simulink model "extControlwithTCP"  (R2019a)
settings: Solver=FixedStepAuto  StartTime=0.0  StopTime=501  FixedStep=0.01  RelTol=1e-3
PreLoadFcn:
  | load('tumbleweed_constants.mat')
InitFcn:
  | coder.extrinsic('controlsolver')
undefined symbols (not defined in the file): d, f, g, Ixx, Iyy, Izz, m, maxr, mf, minr, mu0, R, v_thres, vmax, YY
libraries: instrumentlib x2, simulink x1
settings Model: EnablePacing=on  Creator=racha  LastModifiedBy=racha
settings RTWCC: TargetLang=C++
settings GRTTargetCC: TargetLangStandard=C++03 (ISO)  MultiInstanceERTCode=on  CodeInterfacePackaging=C++ class

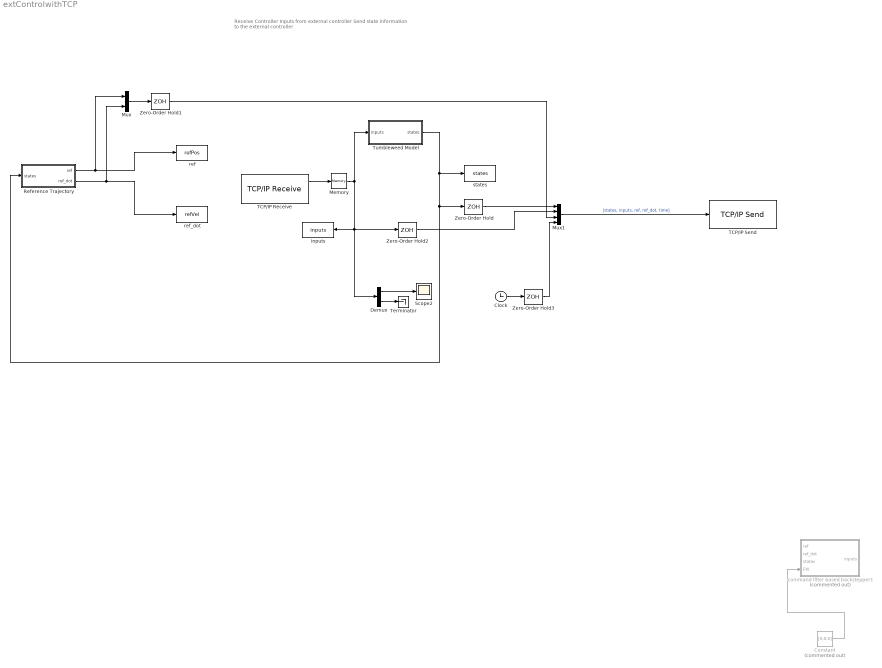
== system extControlwithTCP ==
  note: Receive Controller Inputs from external controller
      | Send state information to the external controller
  Clock : Clock
  Constant : Constant  Commented=on  Value=[0;0;0]
  Demux : Demux  Outputs=[1;17]
  Memory : Memory  InitialCondition=[d/2;-d/2;d/2;-d/2;d/2;-d/2;zeros(12,1)]
  Mux : Mux  Inputs=[3;3]
  Mux1 : Mux  Inputs=[13;18;6;1]
  Reference Trajectory : Subsystem
  Scope2 : Scope
  TCP/IP Receive : instrumentlib/TCP//IP Receive  Priority=4  Host=localhost  Port=54330  DataSize="[18   1]"  EnableBlockingMode=off  Timeout=10  SampleTime=0.01  DataType=double  ByteOrder=LittleEndian  ASCIIFormatting=%f,  Terminator=LF
      settings: SourceProductName=Instrument Control Toolbox
  TCP/IP Send : instrumentlib/TCP//IP Send  Priority=1  Host=localhost  Port=54320  EnableBlockingMode=off  Timeout=10  ByteOrder=LittleEndian  TransferDelay=off
      settings: SourceProductName=Instrument Control Toolbox
  Terminator : Terminator
  Tumbleweed Model : Subsystem
  Zero-Order Hold{,1..3} (4 alike) : ZeroOrderHold  SampleTime=0.01
  command filter based backstepper1 : Subsystem  Commented=on
  inputs : ToWorkspace  VariableName=inputs  SampleTime=-1
      settings: Save2DSignal=2-D array (concatenate along first dimension)
  ref : ToWorkspace  VariableName=refPos  SampleTime=-1
      settings: Save2DSignal=2-D array (concatenate along first dimension)
  ref_dot : ToWorkspace  VariableName=refVel  SampleTime=-1
      settings: Save2DSignal=2-D array (concatenate along first dimension)
  states : ToWorkspace  VariableName=states  SampleTime=-1
      settings: Save2DSignal=2-D array (concatenate along first dimension)
  wires:
  Reference Trajectory/1(ref) -> Mux/1, ref/1
  Reference Trajectory/2("ref_dot ") -> Mux/2, ref_dot/1
  Constant/1 -> command filter based backstepper1/4(FW)
  TCP/IP Receive/1 -> Memory/1
  Mux/1 -> Zero-Order Hold1/1
  Tumbleweed Model/1("states ") -> Reference Trajectory/1(states), Zero-Order Hold/1, states/1
  Zero-Order Hold1/1 -> Mux1/3
  Memory/1 -> Demux/1, inputs/1, Zero-Order Hold2/1, Tumbleweed Model/1(inputs)
  Demux/1 -> Scope2/1
  Demux/2 -> Terminator/1
  Zero-Order Hold/1 -> Mux1/1
  Mux1/1 -> TCP/IP Send/1  "[states, inputs, ref, ref_dot, time]"
  Zero-Order Hold2/1 -> Mux1/2
  Clock/1 -> Zero-Order Hold3/1
  Zero-Order Hold3/1 -> Mux1/4

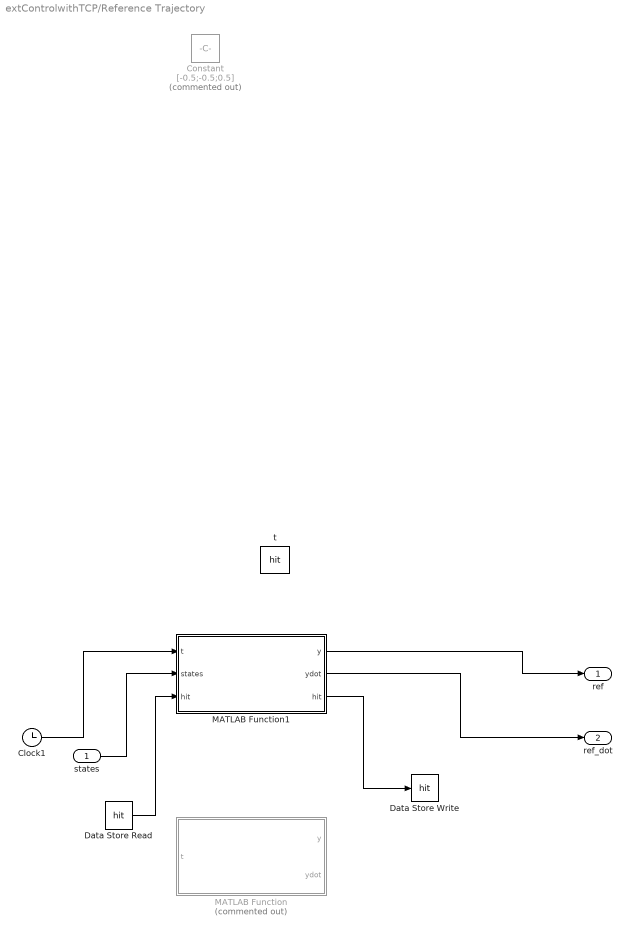
== system extControlwithTCP/Reference Trajectory ==
  states : Inport
  Clock1 : Clock
  Constant : Constant  Commented=on  Value=[-0.5;-0.5;0.5]
  Data Store Read : DataStoreRead  DataStoreName=hit
  Data Store Write : DataStoreWrite  DataStoreName=hit
  MATLAB Function : MATLAB Function  Commented=on  TreatAsAtomicUnit=on
  MATLAB Function1 : MATLAB Function  TreatAsAtomicUnit=on
  t : DataStoreMemory  DataStoreName=hit  ReadBeforeWriteMsg=warning  WriteAfterWriteMsg=warning  WriteAfterReadMsg=warning  ShowAdditionalParam=off
  ref : Outport
  "ref_dot " : Outport  Port=2
  wires:
  MATLAB Function1/2(ydot) -> "ref_dot "/1
  Data Store Read/1 -> MATLAB Function1/3("hit ")
  states/1 -> MATLAB Function1/2(states)
  Clock1/1 -> MATLAB Function1/1(t)
  MATLAB Function1/3(hit) -> Data Store Write/1
  MATLAB Function1/1(y) -> ref/1

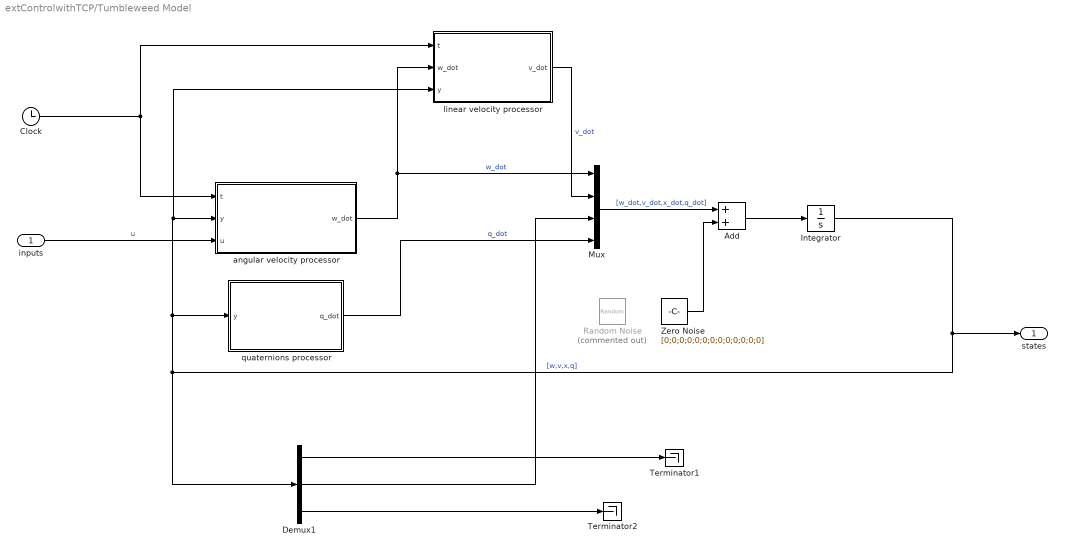
== system extControlwithTCP/Tumbleweed Model ==
  inputs : Inport
  Add : Sum
  Clock : Clock
  Demux1 : Demux  Outputs=[3;3;7]
  Integrator : Integrator  InitialCondition=|
      | [0;
      | 0.001; 0; 0.0005; 0; 0;0;0;R;1;0;0;0]
  Mux : Mux  Inputs=[3;3;3;4]
  Random Noise : RandomNumber  Commented=on  Mean=zeros(13,1)  Variance=[0.1;0.1;0.1;0.1;0.1;0;0.1;0.1;0;0.01;0.01;0.01;0.01]  SampleTime=0.001
  Terminator1 : Terminator
  Terminator2 : Terminator
  Zero Noise : Constant  Value=[0;0;0;0;0;0;0;0;0;0;0;0;0]  OutDataTypeStr=Inherit: Inherit via back propagation
  angular velocity processor : MATLAB Function  TreatAsAtomicUnit=on
  linear velocity processor : MATLAB Function  TreatAsAtomicUnit=on
  quaternions processor : MATLAB Function  TreatAsAtomicUnit=on
  "states " : Outport
  wires:
  Clock/1 -> linear velocity processor/1(t), angular velocity processor/1(t)
  angular velocity processor/1(w_dot) -> Mux/1, linear velocity processor/2(w_dot)  "w_dot"
  quaternions processor/1(q_dot) -> Mux/4  "q_dot"
  inputs/1 -> angular velocity processor/3(u)  "u"
  linear velocity processor/1(v_dot) -> Mux/2  "v_dot"
  Demux1/1 -> Terminator1/1
  Demux1/2 -> Mux/3
  Integrator/1 -> Demux1/1, linear velocity processor/3(y), angular velocity processor/2(y), quaternions processor/1(y), "states "/1  "[w,v,x,q]"
  Demux1/3 -> Terminator2/1
  Mux/1 -> Add/1  "[w_dot,v_dot,x_dot,q_dot]"
  Add/1 -> Integrator/1
  Zero Noise/1 -> Add/2

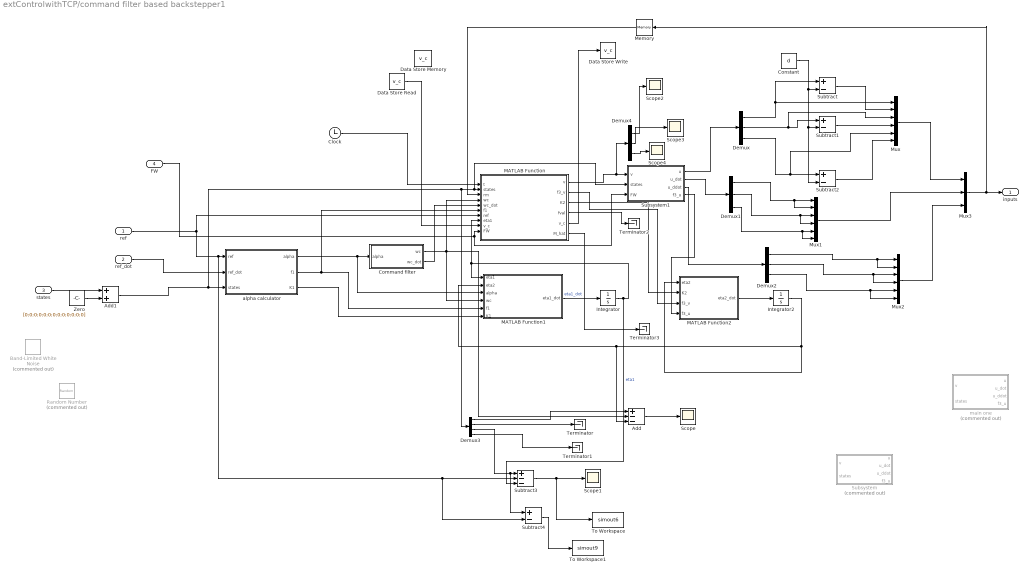
== system extControlwithTCP/command filter based backstepper1 ==
  ref : Inport
  "ref_dot " : Inport  Port=2
  states : Inport  Port=3
  FW : Inport  Port=4
  Add : Sum  Inputs=+--
  Add1 : Sum
  Band-Limited White Noise : simulink/Sources/Band-Limited White Noise  Commented=on  Cov=[0.002;0.002;0.002;0.002;0.002;0.001;0.05;0.05;0.05;0.001;0.001;0.001;0.001]  Ts=0.001  seed=[23340]
  Clock : Clock
  Command filter : Subsystem
  Constant : Constant  Value=d
  Data Store Memory : DataStoreMemory  DataStoreName=v_c  ReadBeforeWriteMsg=warning  WriteAfterWriteMsg=warning  WriteAfterReadMsg=warning  InitialValue=[0.325;0.325;0.325;0]  ShowAdditionalParam=off
  Data Store Read : DataStoreRead  DataStoreName=v_c
  Data Store Write : DataStoreWrite  DataStoreName=v_c
  Demux{,1..2,4} (4 alike) : Demux  Outputs=3
  Demux3 : Demux  Outputs=[3;3;3;4]
  Integrator : Integrator  InitialCondition=[0;0;0]
  Integrator2 : Integrator  InitialCondition=[0;0;0]
  MATLAB Function : MATLAB Function  TreatAsAtomicUnit=on
  MATLAB Function1 : MATLAB Function  TreatAsAtomicUnit=on
  MATLAB Function2 : MATLAB Function  TreatAsAtomicUnit=on
  Memory : Memory  InitialCondition=[d/2;-d/2;d/2;-d/2;d/2;-d/2;0;0;0;0;0;0;0;0;0;0;0;0]
  Mux : Mux  Inputs=6
  Mux1 : Mux  Inputs=6
  Mux2 : Mux  Inputs=6
  Mux3 : Mux  Inputs=3
  Random Number : RandomNumber  Commented=on  Mean=zeros(13,1)  Variance=[0.1;0.1;0.1;0.1;0.1;0.1;0.2;0.2;0.2;0.01;0.01;0.01;0.01]  Seed=randi(1000,13,1)  SampleTime=0.001
  Scope{,1..4} (5 alike) : Scope
  Subsystem : Subsystem  Commented=on
  Subsystem1 : Subsystem
  Subtract{,1..2,4} (4 alike) : Sum  Inputs=+-
  Subtract3 : Sum  Inputs=+--
  Terminator{,1..3} (4 alike) : Terminator
  To Workspace : ToWorkspace  VariableName=simout6  SaveFormat=Timeseries  SampleTime=-1
  To Workspace1 : ToWorkspace  VariableName=simout9  SaveFormat=Timeseries  SampleTime=-1
  Zero : Constant  Value=[0;0;0;0;0;0;0;0;0;0;0;0;0]  OutDataTypeStr=Inherit: Inherit via back propagation
  alpha calculator : MATLAB Function  TreatAsAtomicUnit=on
  main one : Subsystem  Commented=on
  inputs : Outport
  wires:
  alpha calculator/1(alpha) -> Command filter/1(alpha), MATLAB Function1/3(alpha)
  MATLAB Function1/1(eta1_dot) -> Integrator/1  "eta1_dot"
  Integrator/1 -> Subtract3/3, MATLAB Function/8(eta1), MATLAB Function1/1(eta1)  "eta1"
  alpha calculator/2(f1) -> MATLAB Function/6(f1), MATLAB Function1/5(f1)
  alpha calculator/3(K1) -> MATLAB Function1/6(K1)
  ref/1 -> MATLAB Function/7(ref), Subtract4/2, Subtract3/2, alpha calculator/1(ref)
  "ref_dot "/1 -> alpha calculator/2(ref_dot)
  Command filter/2(wc_dot) -> MATLAB Function/5(wc_dot)
  Command filter/1(wc) -> MATLAB Function/4(wc), MATLAB Function1/4(wc), Add/2
  MATLAB Function/1(v) -> Demux4/1, Subsystem1/1(v)
  Subsystem1/1(u) -> Demux/1
  Subsystem1/2(u_dot) -> Demux1/1
  Mux3/1 -> Memory/1, inputs/1
  MATLAB Function/3(K2) -> MATLAB Function2/2(K2)
  MATLAB Function/2(f3_v) -> MATLAB Function2/3(f3_v)
  Subsystem1/4(f3_u) -> MATLAB Function2/4(f3_u)
  MATLAB Function2/1(eta2_dot) -> Integrator2/1
  Integrator2/1 -> MATLAB Function1/2(eta2), Add/3, MATLAB Function2/1(eta2)
  Subsystem1/3(u_ddot) -> Demux2/1
  Demux/3 -> Mux/5, Subtract2/1
  Demux/2 -> Mux/3, Subtract1/1
  Demux/1 -> Mux/1, Subtract/1
  Constant/1 -> Subtract2/2, Subtract1/2, Subtract/2
  Subtract/1 -> Mux/2
  Subtract1/1 -> Mux/4
  Subtract2/1 -> Mux/6
  Mux/1 -> Mux3/1
  Demux1/1 -> Mux1/2, Mux1/1
  Demux1/2 -> Mux1/4, Mux1/3
  Demux1/3 -> Mux1/6, Mux1/5
  Demux2/3 -> Mux2/6, Mux2/5
  Demux2/1 -> Mux2/2, Mux2/1
  Demux2/2 -> Mux2/4, Mux2/3
  Mux1/1 -> Mux3/2
  Mux2/1 -> Mux3/3
  Memory/1 -> MATLAB Function/3(rm)
  Clock/1 -> MATLAB Function/1(t)
  MATLAB Function/4(fval) -> Terminator2/1
  Data Store Read/1 -> MATLAB Function/9("v_c ")
  MATLAB Function/5(v_c) -> Data Store Write/1
  MATLAB Function/6(M_hat) -> Terminator3/1
  Demux3/2 -> Terminator/1
  Demux3/1 -> Add/1
  Add/1 -> Scope/1
  Demux3/4 -> Terminator1/1
  Demux3/3 -> Subtract4/1, Subtract3/1
  Subtract3/1 -> To Workspace/1, Scope1/1
  Add1/1 -> Demux3/1, Subsystem1/2(states), MATLAB Function/2(states), alpha calculator/3(states)
  states/1 -> Add1/1
  Zero/1 -> Add1/2
  FW/1 -> Subsystem1/3(FW), MATLAB Function/10(FW)
  Subtract4/1 -> To Workspace1/1
  Demux4/1 -> Scope2/1
  Demux4/2 -> Scope3/1
  Demux4/3 -> Scope4/1

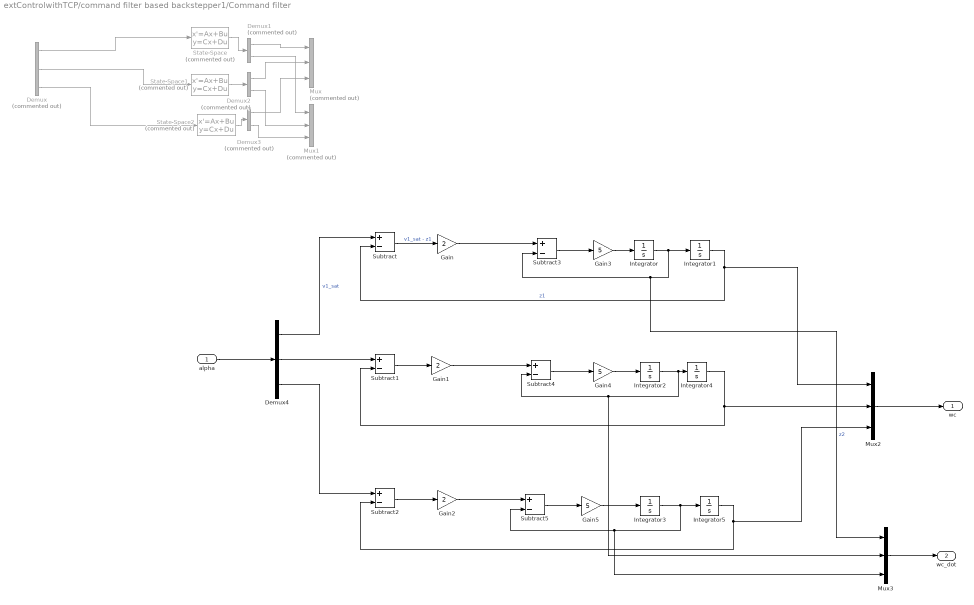
== system extControlwithTCP/command filter based backstepper1/Command filter ==
  alpha : Inport
  Demux : Demux  Commented=on  Outputs=3
  Demux1 : Demux  Commented=on  Outputs=2
  Demux2 : Demux  Commented=on  Outputs=2
  Demux3 : Demux  Commented=on  Outputs=2
  Demux4 : Demux  Outputs=3
  Gain : Gain  Gain=2
  Gain1 : Gain  Gain=2
  Gain2 : Gain  Gain=2
  Gain3 : Gain  Gain=5
  Gain4 : Gain  Gain=5
  Gain5 : Gain  Gain=5
  Integrator{,1..5} (6 alike) : Integrator
  Mux : Mux  Commented=on  Inputs=3
  Mux1 : Mux  Commented=on  Inputs=3
  Mux2 : Mux  Inputs=3
  Mux3 : Mux  Inputs=3
  State-Space : StateSpace  Commented=on  A=[0, 10; -2*0.8*10, -10]  B=[0;20]  C=[1,0;0,1]  D=[0;0]  InitialCondition=[0;0]
  State-Space1 : StateSpace  Commented=on  A=[0, 10; -2*0.8*10, -10]  B=[0;20]  C=[1,0;0,1]  D=[0;0]  InitialCondition=[0;0]
  State-Space2 : StateSpace  Commented=on  A=[0, 10; -2*0.8*10, -10]  B=[0;5]  C=[1,0;0,1]  D=[0;0]  InitialCondition=[0;0]
  Subtract{,1..5} (6 alike) : Sum  Inputs=+-
  wc : Outport
  wc_dot : Outport  Port=2
  wires:
  State-Space/1 -> Demux1/1
  Demux/1 -> State-Space/1
  Demux/2 -> State-Space1/1
  Demux/3 -> State-Space2/1
  State-Space1/1 -> Demux2/1
  Demux2/1 -> Mux/2
  State-Space2/1 -> Demux3/1
  Demux1/1 -> Mux/1
  Demux3/1 -> Mux/3
  Demux1/2 -> Mux1/1
  Demux2/2 -> Mux1/2
  Demux3/2 -> Mux1/3
  Mux2/1 -> wc/1
  alpha/1 -> Demux4/1
  Demux4/1 -> Subtract/1  "v1_sat"
  Gain3/1 -> Integrator/1
  Subtract/1 -> Gain/1  "v1_sat - z1"
  Subtract5/1 -> Gain5/1
  Gain/1 -> Subtract3/1
  Subtract2/1 -> Gain2/1
  Integrator2/1 -> Mux3/2, Subtract4/2, Integrator4/1
  Gain4/1 -> Integrator2/1
  Subtract1/1 -> Gain1/1
  Subtract3/1 -> Gain3/1
  Subtract4/1 -> Gain4/1
  Gain5/1 -> Integrator3/1
  Integrator/1 -> Integrator1/1, Mux3/1, Subtract3/2  "z2"
  Integrator5/1 -> Subtract2/2, Mux2/3
  Mux3/1 -> wc_dot/1
  Gain1/1 -> Subtract4/1
  Gain2/1 -> Subtract5/1
  Integrator4/1 -> Subtract1/2, Mux2/2
  Integrator3/1 -> Mux3/3, Subtract5/2, Integrator5/1
  Integrator1/1 -> Subtract/2, Mux2/1  "z1"
  Demux4/2 -> Subtract1/1
  Demux4/3 -> Subtract2/1

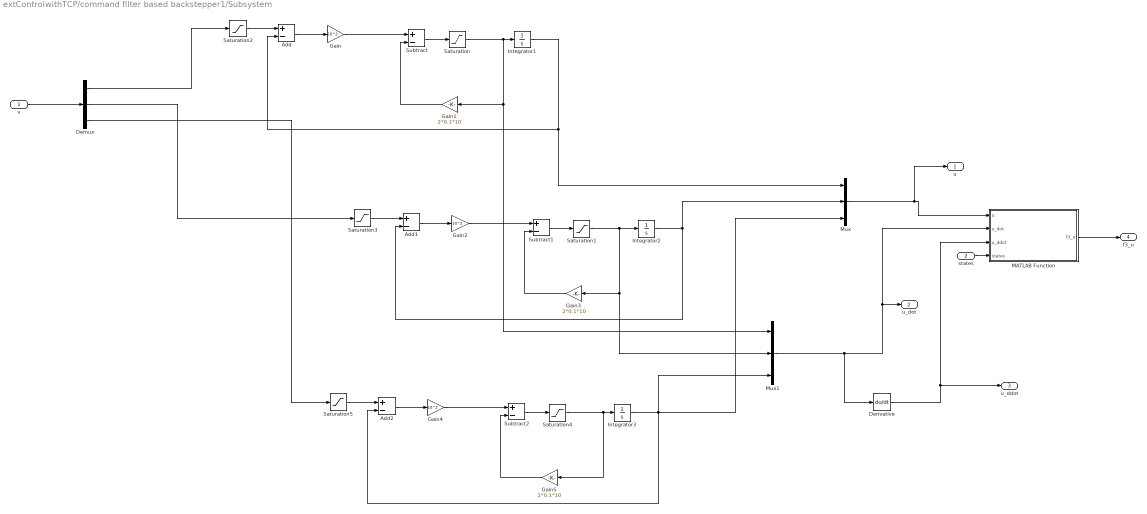
== system extControlwithTCP/command filter based backstepper1/Subsystem ==
  v : Inport
  states : Inport  Port=2
  Add : Sum  Inputs=+-
  Add1 : Sum  Inputs=+-
  Add2 : Sum  Inputs=+-
  Demux : Demux  Outputs=3
  Derivative : Derivative  CoefficientInTFapproximation=0
  Gain : Gain  Gain=10^2
  Gain1 : Gain  Gain=2*0.1*10
  Gain2 : Gain  Gain=10^2
  Gain3 : Gain  Gain=2*0.1*10
  Gain4 : Gain  Gain=10^2
  Gain5 : Gain  Gain=2*0.1*10
  Integrator1 : Integrator  InitialCondition=d/2
  Integrator2 : Integrator  InitialCondition=d/2
  Integrator3 : Integrator  InitialCondition=d/2
  MATLAB Function : MATLAB Function  TreatAsAtomicUnit=on
  Mux : Mux  Inputs=3
  Mux1 : Mux  Inputs=3
  Saturation : Saturate  UpperLimit=vmax  LowerLimit=-vmax
  Saturation1 : Saturate  UpperLimit=vmax  LowerLimit=-vmax
  Saturation2 : Saturate  UpperLimit=maxr  LowerLimit=minr
  Saturation3 : Saturate  UpperLimit=maxr  LowerLimit=minr
  Saturation4 : Saturate  UpperLimit=vmax  LowerLimit=-vmax
  Saturation5 : Saturate  UpperLimit=maxr  LowerLimit=minr
  Subtract : Sum  Inputs=+-
  Subtract1 : Sum  Inputs=+-
  Subtract2 : Sum  Inputs=+-
  u : Outport
  u_dot : Outport  Port=2
  u_ddot : Outport  Port=3
  f3_u : Outport  Port=4
  wires:
  Saturation/1 -> Mux1/1, Gain1/1, Integrator1/1
  Demux/1 -> Saturation2/1
  Gain1/1 -> Subtract/2
  Gain/1 -> Subtract/1
  Subtract/1 -> Saturation/1
  Integrator1/1 -> Mux/1, Add/2
  Add/1 -> Gain/1
  Saturation2/1 -> Add/1
  v/1 -> Demux/1
  Saturation1/1 -> Integrator2/1, Mux1/2, Gain3/1
  Saturation3/1 -> Add1/1
  Add1/1 -> Gain2/1
  Integrator2/1 -> Add1/2, Mux/2
  Gain2/1 -> Subtract1/1
  Gain3/1 -> Subtract1/2
  Demux/2 -> Saturation3/1
  Subtract1/1 -> Saturation1/1
  Saturation4/1 -> Gain5/1, Integrator3/1
  Saturation5/1 -> Add2/1
  Add2/1 -> Gain4/1
  Integrator3/1 -> Mux1/3, Add2/2, Mux/3
  Gain4/1 -> Subtract2/1
  Gain5/1 -> Subtract2/2
  Demux/3 -> Saturation5/1
  Subtract2/1 -> Saturation4/1
  Mux1/1 -> Derivative/1, u_dot/1, MATLAB Function/2(u_dot)
  Mux/1 -> u/1, MATLAB Function/1(u)
  Derivative/1 -> MATLAB Function/3(u_ddot), u_ddot/1
  states/1 -> MATLAB Function/4(states)
  MATLAB Function/1(f3_u) -> f3_u/1

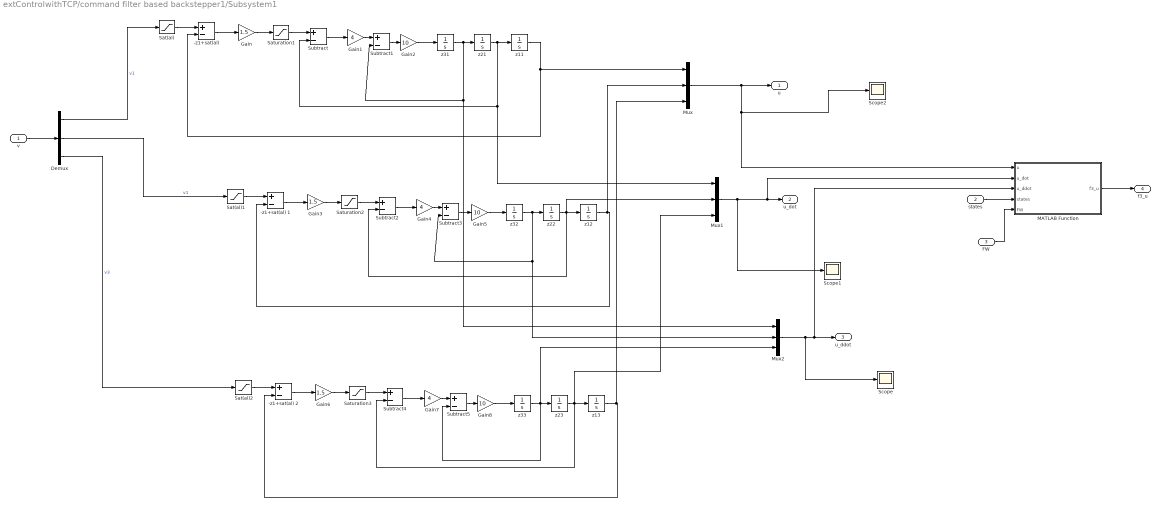
== system extControlwithTCP/command filter based backstepper1/Subsystem1 ==
  v : Inport
  states : Inport  Port=2
  FW : Inport  Port=3
  "-z1+sat(al) " : Sum  Inputs=+-
  -z1+sat(al) 1 : Sum  Inputs=+-
  -z1+sat(al) 2 : Sum  Inputs=+-
  Demux : Demux  Outputs=3
  Gain : Gain  Gain=1.5
  Gain1 : Gain  Gain=4
  Gain2 : Gain  Gain=10
  Gain3 : Gain  Gain=1.5
  Gain4 : Gain  Gain=4
  Gain5 : Gain  Gain=10
  Gain6 : Gain  Gain=1.5
  Gain7 : Gain  Gain=4
  Gain8 : Gain  Gain=10
  MATLAB Function : MATLAB Function  TreatAsAtomicUnit=on
  Mux : Mux  Inputs=3
  Mux1 : Mux  Inputs=3
  Mux2 : Mux  Inputs=3
  Sat(al) : Saturate  UpperLimit=maxr  LowerLimit=minr  LinearizeAsGain=off
  Sat(al)1 : Saturate  UpperLimit=maxr  LowerLimit=minr  LinearizeAsGain=off
  Sat(al)2 : Saturate  UpperLimit=maxr  LowerLimit=minr
  Saturation1 : Saturate  UpperLimit=vmax  LowerLimit=-vmax
  Saturation2 : Saturate  UpperLimit=vmax  LowerLimit=-vmax
  Saturation3 : Saturate  UpperLimit=vmax  LowerLimit=-vmax
  Scope : Scope
  Scope1 : Scope
  Scope2 : Scope
  Subtract{,1..5} (6 alike) : Sum  Inputs=+-
  z11 : Integrator  InitialCondition=d/2
  z12 : Integrator  InitialCondition=d/2
  z13 : Integrator  InitialCondition=d/2
  z{21..23,31..33} (6 alike) : Integrator
  u : Outport
  u_dot : Outport  Port=2
  u_ddot : Outport  Port=3
  f3_u : Outport  Port=4
  wires:
  Saturation1/1 -> Subtract/1
  Subtract/1 -> Gain1/1
  Sat(al)/1 -> "-z1+sat(al) "/1
  Gain/1 -> Saturation1/1
  "-z1+sat(al) "/1 -> Gain/1
  z11/1 -> Mux/1, "-z1+sat(al) "/2
  Subtract1/1 -> Gain2/1
  z31/1 -> Mux2/1, Subtract1/2, z21/1
  Gain1/1 -> Subtract1/1
  Gain2/1 -> z31/1
  Demux/1 -> Sat(al)/1  "v1"
  v/1 -> Demux/1
  Demux/3 -> Sat(al)2/1  "v3"
  Gain5/1 -> z32/1
  Gain4/1 -> Subtract3/1
  Subtract3/1 -> Gain5/1
  z32/1 -> Mux2/2, Subtract3/2, z22/1
  Demux/2 -> Sat(al)1/1  "v1"
  z22/1 -> Mux1/2, Subtract2/2, z12/1
  z12/1 -> Mux/2, -z1+sat(al) 1/2
  -z1+sat(al) 1/1 -> Gain3/1
  Gain3/1 -> Saturation2/1
  Sat(al)1/1 -> -z1+sat(al) 1/1
  Saturation2/1 -> Subtract2/1
  Subtract2/1 -> Gain4/1
  Gain8/1 -> z33/1
  Gain7/1 -> Subtract5/1
  Subtract5/1 -> Gain8/1
  z33/1 -> Mux2/3, Subtract5/2, z23/1
  z23/1 -> Mux1/3, Subtract4/2, z13/1
  z13/1 -> Mux/3, -z1+sat(al) 2/2
  -z1+sat(al) 2/1 -> Gain6/1
  Gain6/1 -> Saturation3/1
  Sat(al)2/1 -> -z1+sat(al) 2/1
  Saturation3/1 -> Subtract4/1
  Subtract4/1 -> Gain7/1
  z21/1 -> Mux1/1, Subtract/2, z11/1
  MATLAB Function/1(f3_u) -> f3_u/1
  Mux2/1 -> Scope/1, MATLAB Function/3(u_ddot), u_ddot/1
  Mux/1 -> Scope2/1, MATLAB Function/1(u), u/1
  states/1 -> MATLAB Function/4(states)
  Mux1/1 -> Scope1/1, MATLAB Function/2(u_dot), u_dot/1
  FW/1 -> MATLAB Function/5(FW)

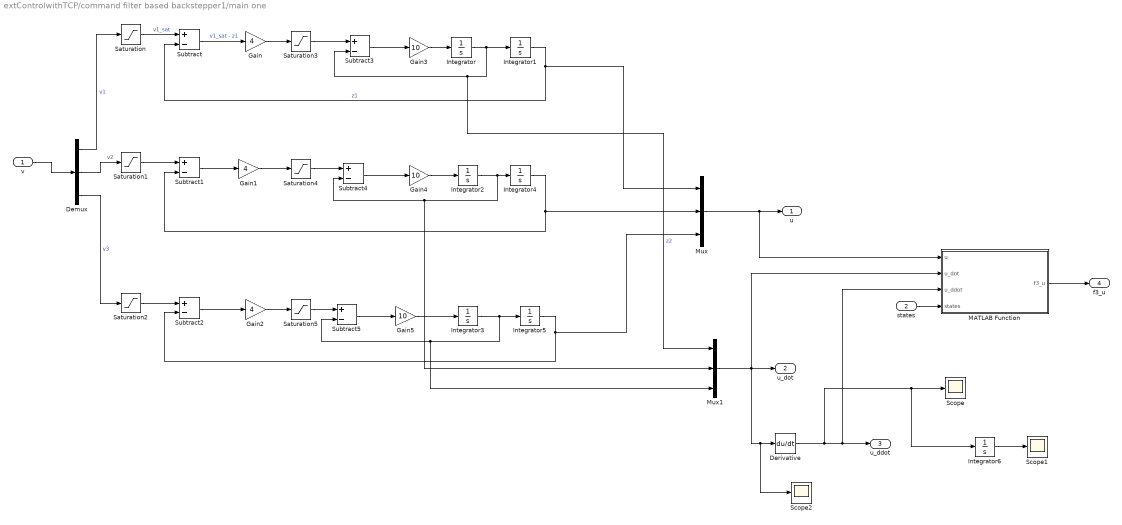
== system extControlwithTCP/command filter based backstepper1/main one ==
  v : Inport
  states : Inport  Port=2
  Demux : Demux  Outputs=3
  Derivative : Derivative  CoefficientInTFapproximation=0
  Gain : Gain  Gain=4
  Gain1 : Gain  Gain=4
  Gain2 : Gain  Gain=4
  Gain3 : Gain  Gain=10
  Gain4 : Gain  Gain=10
  Gain5 : Gain  Gain=10
  Integrator{,2..3,6} (4 alike) : Integrator
  Integrator1 : Integrator  InitialCondition=d/2
  Integrator4 : Integrator  InitialCondition=d/2
  Integrator5 : Integrator  InitialCondition=d/2
  MATLAB Function : MATLAB Function  TreatAsAtomicUnit=on
  Mux : Mux  Inputs=3
  Mux1 : Mux  Inputs=3
  Saturation : Saturate  UpperLimit=maxr  LowerLimit=minr
  Saturation1 : Saturate  UpperLimit=maxr  LowerLimit=minr
  Saturation2 : Saturate  UpperLimit=maxr  LowerLimit=minr
  Saturation3 : Saturate  UpperLimit=vmax  LowerLimit=-vmax
  Saturation4 : Saturate  UpperLimit=vmax  LowerLimit=-vmax
  Saturation5 : Saturate  UpperLimit=vmax  LowerLimit=-vmax
  Scope : Scope
  Scope1 : Scope
  Scope2 : Scope
  Subtract{,1..5} (6 alike) : Sum  Inputs=+-
  u : Outport
  u_dot : Outport  Port=2
  u_ddot : Outport  Port=3
  f3_u : Outport  Port=4
  wires:
  v/1 -> Demux/1
  Demux/1 -> Saturation/1  "v1"
  Demux/2 -> Saturation1/1  "v2"
  Demux/3 -> Saturation2/1  "v3"
  Saturation/1 -> Subtract/1  "v1_sat"
  Saturation1/1 -> Subtract1/1
  Saturation2/1 -> Subtract2/1
  Subtract/1 -> Gain/1  "v1_sat - z1"
  Subtract1/1 -> Gain1/1
  Subtract2/1 -> Gain2/1
  Gain/1 -> Saturation3/1
  Gain1/1 -> Saturation4/1
  Gain2/1 -> Saturation5/1
  Saturation3/1 -> Subtract3/1
  Saturation4/1 -> Subtract4/1
  Saturation5/1 -> Subtract5/1
  Subtract3/1 -> Gain3/1
  Subtract4/1 -> Gain4/1
  Subtract5/1 -> Gain5/1
  Gain3/1 -> Integrator/1
  Integrator/1 -> Integrator1/1, Mux1/1, Subtract3/2  "z2"
  Integrator1/1 -> Subtract/2, Mux/1  "z1"
  Gain4/1 -> Integrator2/1
  Gain5/1 -> Integrator3/1
  Integrator2/1 -> Mux1/2, Subtract4/2, Integrator4/1
  Integrator4/1 -> Subtract1/2, Mux/2
  Integrator5/1 -> Subtract2/2, Mux/3
  Mux/1 -> MATLAB Function/1(u), u/1
  Integrator3/1 -> Mux1/3, Subtract5/2, Integrator5/1
  Derivative/1 -> Integrator6/1, Scope/1, MATLAB Function/3(u_ddot), u_ddot/1
  Mux1/1 -> MATLAB Function/2(u_dot), Scope2/1, Derivative/1, u_dot/1
  states/1 -> MATLAB Function/4(states)
  MATLAB Function/1(f3_u) -> f3_u/1
  Integrator6/1 -> Scope1/1

== matlab function extControlwithTCP/Reference Trajectory/MATLAB Function ==
  data: t input; y output; ydot output; R parameter
function [y, ydot] = reference_trajectory_generator(t,R)
% xr = 0.2*t;
% yr = 4*sin(0.2/3*t);
% zr = 0.5;
% 
% xr_dot = 0.2;
% yr_dot = 4*cos(0.2/3*t)*(0.3/3);
% zr_dot = 0;
% xr = 30*cos(0.1/3*t);
% yr = 30*sin(0.1/3*t);
% zr = R;
% xr_dot = -30*sin(0.1/3*t)*(0.1/3);
% yr_dot = 30*cos(0.1/3*t)*(0.1/3);
% zr_dot = 0;
% 
% y = [xr;yr;zr];
% ydot = [xr_dot; yr_dot; zr_dot];

% xr = 5*cos(0.2/3*t);
% yr = 5*sin(0.2/3*t);
% zr = 0.5;
% 
% xr_dot = -5*sin(0.2/3*t)*0.2/3;
% yr_dot = 5*cos(0.2/3*t)*(0.2/3);
% zr_dot = 0;

if(t<50)
    xr = 0.2*t;
    yr = 0;
    zr = 0.5;
    xr_dot = 0.2;
    yr_dot = 0;
    zr_dot = 0;
elseif(t>50 && t<100)
        xr = 10;
    yr = 0.2*(t-50);
    zr = 0.5;
    xr_dot = 0;
    yr_dot = 0.2;
    zr_dot = 0;
elseif(t>100 && t<150)
        xr = 10 - 0.2*(t-100) ;
    yr = 10;
    zr = 0.5;
    xr_dot = -0.2;
    yr_dot = 0;
    zr_dot = 0;
elseif(t>150 && t<200)
        xr = 0;
    yr = 10 - 0.2*(t-150);
    zr = 0.5;
    xr_dot = 0;
    yr_dot = -0.2;
    zr_dot = 0;
else
 xr = 0;
 yr = 0;
 zr = 0.5;
 
 xr_dot = 0;
 yr_dot = 0;
 zr_dot = 0;
end

y = [xr;yr;zr];
ydot = [xr_dot; yr_dot; zr_dot];

end

== matlab function extControlwithTCP/Reference Trajectory/MATLAB Function1 ==
  data: t input; y output; ydot output; states input; hit input; hit output; R parameter
function [y, ydot,hit] = reference_trajectory_generator(t,states,hit,R)

% xr = 100;
%  yr = 0;
%  zr = R;
%         
%  
% xr_dot = 0;
% yr_dot = 0;
% zr_dot = 0;
% 
% if hit == 0
% if t ~= 0    
%  xr = 10;
%  yr = 0;
%  zr = R;
%         
%  
% xr_dot = 0;
% yr_dot = 0;
% zr_dot = 0;
% else
%      xr = 0;
%  yr = 0;
%  zr = R;
%         
%  
% xr_dot = 0;
% yr_dot = 0;
% zr_dot = 0;
% end
% elseif hit == 1
%        xr = 10;
%  yr = 10;
%  zr = R;
%         
%  
% xr_dot = 0;
% yr_dot = 0;
% zr_dot = 0;
% elseif hit == 2
%      xr =0;
%  yr = 10;
%  zr = R;       
% % 
% xr_dot = 0;
% yr_dot = 0;
% zr_dot = 0;
% elseif hit == 3
%        xr = 0;
%  yr = 0;
%  zr = R;
%         
% 
% xr_dot = 0;
% yr_dot = 0;
% zr_dot = 0;
% else
%            xr = 0;
%  yr = 0;
%  zr = R;
%         
% 
% xr_dot = 0;
% yr_dot = 0;
% zr_dot = 0;
% end
% 
% if hit == 0 && (t ~=0 )&& norm([states(7)- xr;states(8)- yr])<=0.3
%     hit = 1;
% elseif hit == 1 && norm([states(7)- xr;states(8)- yr])<=0.3
%     hit = 2;
% elseif hit == 2 && norm([states(7)- xr;states(8)- yr])<=0.3
%     hit = 3;
% elseif hit == 3 && norm([states(7)- xr;states(8)- yr])<=0.3
%     hit = 4;
% else
%     hit = hit;
% end

% xr = 0.25*t;
% yr = 4*sin(0.25/3*t);
% zr = 0.5;
% 
% xr_dot = 0.25;
% yr_dot = 4*cos(0.25/3*t)*(0.25/3);
% zr_dot = 0;

% 
 xr = 5*cos(0.2/3*t);
yr = 5*sin(0.2/3*t);
zr = 0.5;

xr_dot = -5*sin(0.2/3*t)*0.2/3;
yr_dot = 5*cos(0.2/3*t)*(0.2/3);
zr_dot = 0;

% xr = 30*cos(0.062/3*t);
% yr = 30*sin(0.062/3*t);
% zr = R;
% xr_dot = -30*sin(0.062/3*t)*(0.062/3);
% yr_dot = 30*cos(0.062/3*t)*(0.062/3);
% zr_dot = 0;


y = [xr;yr;zr];
ydot = [xr_dot; yr_dot; zr_dot];

end

== matlab function extControlwithTCP/Tumbleweed Model/angular velocity processor ==
  data: t input; y input; u input; w_dot output; R parameter; g parameter; Ixx parameter; Iyy parameter; Izz parameter; m parameter; mf parameter; mu0 parameter; v_thres parameter; d parameter; YY parameter
function w_dot = angular_velocity_processor(t, y,u, R, g, Ixx, Iyy, Izz, m, mf, mu0, v_thres, d, YY)
%y = [wx, wy, wz,u,v,w, x,y,z,q0,q1,q2,q3];
%u =[r_m1T,r_m2T,r_m3T,r_m4T,r_m5T,r_m6T,T_v_m1T,T_v_m2T,T_v_m3T,T_v_m4T,T_v_m5T,T_v_m6T,...
%T_a_m1T,T_a_m2T,T_a_m3T,T_a_m4T,T_a_m5T,T_a_m6T];

I_T = [Ixx,0,0;0,Iyy,0;0,0,Izz];
r_m1T = [u(1);0;0]; T_v_m1T = [u(7);0;0]; T_a_m1T = [u(13);0;0];
r_m2T = [u(2);0;0]; T_v_m2T = [u(8);0;0]; T_a_m2T = [u(14);0;0];
r_m3T = [0;u(3);0]; T_v_m3T = [0;u(9);0]; T_a_m3T = [0;u(15);0];
r_m4T = [0;u(4);0]; T_v_m4T = [0;u(10);0]; T_a_m4T = [0;u(16);0];
r_m5T = [0;0;u(5)]; T_v_m5T = [0;0;u(11)]; T_a_m5T = [0;0;u(17)];
r_m6T = [0;0;u(6)]; T_v_m6T = [0;0;u(12)]; T_a_m6T = [0;0;u(18)];
r_CMT = m*(r_m1T + r_m2T + r_m3T + r_m4T + r_m5T + r_m6T)/(6*m+mf);
T_v_CMT = m*(T_v_m1T + T_v_m2T + T_v_m3T + T_v_m4T + T_v_m5T + T_v_m6T)/(6*m+mf);
T_a_CMT = m*(T_a_m1T + T_a_m2T + T_a_m3T + T_a_m4T + T_a_m5T + T_a_m6T)/(6*m+mf);
r_CMTx = Vx(r_CMT);r_m1Tx = Vx(r_m1T);r_m2Tx = Vx(r_m2T);r_m3Tx = Vx(r_m3T);
r_m4Tx = Vx(r_m4T);r_m5Tx = Vx(r_m5T);r_m6Tx = Vx(r_m6T);
q0 = y(10);q1=y(11);q2=y(12);q3=y(13);
T_c_O = [q0^2 + q1^2 - q2^2 - q3^2, 2*(q1*q2 + q0*q3), 2*(q1*q3 - q0*q2);...
       2*(q1*q2 - q0*q3), q0^2 - q1^2 + q2^2 - q3^2, 2*(q2*q3 + q0*q1);...
       2*(q1*q3 + q0*q2), 2*(q2*q3 - q0*q1), q0^2 - q1^2 - q2^2 + q3^2];
O_c_T = transpose(T_c_O);  
r_PT = [0;0;-R];
r_PTx = Vx([0;0;-R]);
O_w_T = [y(1);y(2);y(3)]; O_w_Tx =Vx(O_w_T);

O_vel_TO = Vx(O_c_T*O_w_T)*[0;0;R];
u_TO = O_vel_TO(1);
v_TO = O_vel_TO(2);

murr = mu0*tanh((u_TO^2 + v_TO^2)/v_thres); 
roll_rest_coeff = [1,0,-murr*u_TO/sqrt(u_TO^2 + v_TO^2);0,1,-murr*v_TO/sqrt(u_TO^2 + v_TO^2);0,0,1];
FG = [0;0;-(mf+6*m)*g];
FR  = -murr*norm(FG)/sqrt(u_TO^2 + v_TO^2)*[u_TO; v_TO; 0];

eps = 0.025;
N = norm(FG'*[0;0;1]);
f = 0.5;
OwTz = (O_c_T*O_w_T)'*[0;0;1];
if(OwTz == 0)
    MzT = [0;0;0];
else
MzT = [0;0;-3*pi*N*f*eps*OwTz/(16*norm(OwTz))];%-mu*N*[0;0;1];
end

Amat = I_T + (mf + 6*m)*r_CMTx*T_c_O*r_PTx*O_c_T - m*r_m1Tx*r_m1Tx - m*r_m2Tx*r_m2Tx...
       - m*r_m3Tx*r_m3Tx - m*r_m4Tx*r_m4Tx - m*r_m5Tx*r_m5Tx - m*r_m6Tx*r_m6Tx...
       - (mf + 6*m)*Vx(T_c_O*r_PT)*Vx(T_c_O*r_PT) + (mf + 6*m)*Vx(T_c_O*r_PT)*r_CMTx;

Bvec = -cross(O_w_T,I_T*O_w_T) - m*cross(r_m1T,2*O_w_Tx*T_v_m1T + O_w_Tx*O_w_Tx*r_m1T)...
       - m*r_m2Tx*(T_a_m2T + 2*O_w_Tx*T_v_m2T + O_w_Tx*O_w_Tx*r_m2T)...
       - m*r_m3Tx*(T_a_m3T + 2*O_w_Tx*T_v_m3T + O_w_Tx*O_w_Tx*r_m3T)...
       - m*r_m4Tx*(T_a_m4T + 2*O_w_Tx*T_v_m4T + O_w_Tx*O_w_Tx*r_m4T)...
       - m*r_m5Tx*(T_a_m5T + 2*O_w_Tx*T_v_m5T + O_w_Tx*O_w_Tx*r_m5T)...
       - m*r_m6Tx*(T_a_m6T + 2*O_w_Tx*T_v_m6T + O_w_Tx*O_w_Tx*r_m6T)...
       + r_CMTx*T_c_O*FG + (mf + 6*m)*cross(T_c_O*r_PT, T_a_CMT + ...
         2*O_w_Tx*T_v_CMT + O_w_Tx*O_w_Tx*r_CMT) - T_c_O*cross(r_PT, FG) ...
         - T_c_O*cross(r_PT, FR) + T_c_O*MzT;
   if t == 8.3
       disp(t);
   end
w_dot = inv(Amat)*Bvec;

== matlab function extControlwithTCP/Tumbleweed Model/quaternions processor ==
  data: y input; q_dot output; R parameter; g parameter; Ixx parameter; Iyy parameter; Izz parameter; m parameter; mf parameter; mu0 parameter; v_thres parameter; d parameter; YY parameter
function q_dot = quaternions_processor(y, R, g, Ixx, Iyy, Izz, m, mf, mu0, v_thres, d, YY)
wx = y(1); wy = y(2); wz = y(3);
q0 = y(10); q1=y(11); q2 = y(12); q3 = y(13);
q_dot = ...
      1/2*[0,-wx,-wy,-wz; wx,0,wz,-wy; wy,-wz,0,wx; ...
      wz,wy,-wx,0]*[q0;q1;q2;q3]+YY/2*(1 - [q0,q1,q2,q3]*...
      [q0;q1;q2;q3])*[q0;q1;q2;q3];

end

== matlab function extControlwithTCP/Tumbleweed Model/linear velocity processor ==
  data: t input; w_dot input; y input; v_dot output; R parameter; g parameter; Ixx parameter; Iyy parameter; Izz parameter; m parameter; mf parameter; mu0 parameter; v_thres parameter; d parameter; YY parameter
function v_dot = linear_velocity_processor(t,w_dot,y, R, g, Ixx, Iyy, Izz, m, mf, mu0, v_thres, d, YY)
%[1;1; 1;0.855496810139384;0.308982518346800;0.188118491654147;-0.370482043830479]
v_dot = zeros(3,1);
O_al_T = [w_dot(1);w_dot(2);w_dot(3)]; 
q0 = y(10);q1=y(11);q2=y(12);q3=y(13);
T_c_O = [q0^2 + q1^2 - q2^2 - q3^2, 2*(q1*q2 + q0*q3), 2*(q1*q3 - q0*q2);...
       2*(q1*q2 - q0*q3), q0^2 - q1^2 + q2^2 - q3^2, 2*(q2*q3 + q0*q1);...
       2*(q1*q3 + q0*q2), 2*(q2*q3 - q0*q1), q0^2 - q1^2 - q2^2 + q3^2];
O_c_T = transpose(T_c_O);
if(t == 3)
    disp(t)
end

v = Vx(O_c_T*O_al_T)*[0;0;R];
v_dot(1,1) = v(1);
v_dot(2,1) = v(2);
v_dot(3,1) = v(3);
end

== matlab function extControlwithTCP/command filter based backstepper1/MATLAB Function ==
  data: t input; states input; rm input; v output size=3; wc input size=3; wc_dot input size=3; f1 input; ref input size=3; eta1 input; v_c input; FW input; v_thres parameter; d parameter; R parameter; mu0 parameter; mf parameter; m parameter; Izz parameter; Iyy parameter; Ixx parameter; g parameter; f3_v output size=3; K2 output size=[3,3]; fval output size=1; v_c output; M_hat output size=[3,3]; minr parameter size=1; maxr parameter size=1; vmax parameter
function [v,f3_v, K2,fval,v_c,M_hat]    = v_calculator(t, states, rm, wc, wc_dot, f1, ref, eta1, v_c,FW,v_thres, d, R, mu0, mf, m, Izz, Iyy, Ixx, g,minr, maxr, vmax)
x = [states(7);states(8);states(9)];
O_w_T = [states(1);states(2);states(3)]; 
if t ==55
    disp(t)
end
K2 = 0.5*eye(3);
ts = 0.01;
v = zeros(3,1);
fval = 0;
if mod(t,0.1) == 0
lhs = wc_dot - K2*(O_w_T - wc) - (f1.')*(x - ref -eta1);
%FW = [0;0;0];
[v, fval] = controlsolver(ts, lhs, states, rm, FW,g, Ixx, Iyy, Izz, m, mf, mu0, R, d, v_thres, minr, maxr);


else
    v = v_c(1:3,1);
    fval = v_c(4,1);
end
v_c = [v;fval];

I_T = [Ixx,0,0;0,Iyy,0;0,0,Izz];
r_m1T = [v(1);0;0];             T_v_m1T = [rm(7);0;0]; T_a_m1T = [rm(13);0;0];
r_m2T = [-(d - v(1));0;0];      T_v_m2T = [rm(8);0;0]; T_a_m2T = [rm(14);0;0];
r_m3T = [0;v(2);0];             T_v_m3T = [0;rm(9);0]; T_a_m3T = [0;rm(15);0];
r_m4T = [0;-(d - v(2));0];      T_v_m4T = [0;rm(10);0]; T_a_m4T = [0;rm(16);0];
r_m5T = [0;0;v(3)];             T_v_m5T = [0;0;rm(11)]; T_a_m5T = [0;0;rm(17)];
r_m6T = [0;0;-(d - v(3))];      T_v_m6T = [0;0;rm(12)]; T_a_m6T = [0;0;rm(18)];
r_CMT = m*(r_m1T + r_m2T + r_m3T + r_m4T + r_m5T + r_m6T)/(6*m+mf);
T_v_CMT = m*(T_v_m1T + T_v_m2T + T_v_m3T + T_v_m4T + T_v_m5T + T_v_m6T)/(6*m+mf);
T_a_CMT = m*(T_a_m1T + T_a_m2T + T_a_m3T + T_a_m4T + T_a_m5T + T_a_m6T)/(6*m+mf);
r_CMTx = Vx(r_CMT);r_m1Tx = Vx(r_m1T);r_m2Tx = Vx(r_m2T);r_m3Tx = Vx(r_m3T);
r_m4Tx = Vx(r_m4T);r_m5Tx = Vx(r_m5T);r_m6Tx = Vx(r_m6T);
q0 = states(10);q1=states(11);q2=states(12);q3=states(13);
T_c_O = [q0^2 + q1^2 - q2^2 - q3^2, 2*(q1*q2 + q0*q3), 2*(q1*q3 - q0*q2);...
       2*(q1*q2 - q0*q3), q0^2 - q1^2 + q2^2 - q3^2, 2*(q2*q3 + q0*q1);...
       2*(q1*q3 + q0*q2), 2*(q2*q3 - q0*q1), q0^2 - q1^2 - q2^2 + q3^2];
O_c_T = transpose(T_c_O);  
r_PT = [0;0;-R];
r_PTx = Vx([0;0;-R]);
O_w_T = [states(1);states(2);states(3)]; O_w_Tx =Vx(O_w_T);

O_vel_TO = Vx(O_c_T*O_w_T)*[0;0;R];
u_TO = O_vel_TO(1);
v_TO = O_vel_TO(2);

murr = mu0*tanh((u_TO^2 + v_TO^2)/v_thres); 
roll_rest_coeff = [1,0,-murr*u_TO/sqrt(u_TO^2 + v_TO^2);0,1,-murr*v_TO/sqrt(u_TO^2 + v_TO^2);0,0,1];
FG = [0;0;-(mf+6*m)*g];
FR  = -murr*norm(FG)/sqrt(u_TO^2 + v_TO^2)*[u_TO; v_TO; 0];

Amat = I_T + (mf + 6*m)*r_CMTx*T_c_O*r_PTx*O_c_T - m*r_m1Tx*r_m1Tx - m*r_m2Tx*r_m2Tx...
       - m*r_m3Tx*r_m3Tx - m*r_m4Tx*r_m4Tx - m*r_m5Tx*r_m5Tx - m*r_m6Tx*r_m6Tx...
       - (mf + 6*m)*Vx(T_c_O*r_PT)*Vx(T_c_O*r_PT) + (mf + 6*m)*Vx(T_c_O*r_PT)*r_CMTx;
  %some mistakes here. check again 
Bvec = -cross(O_w_T,I_T*O_w_T) - m*cross(r_m1T,2*O_w_Tx*T_v_m1T + O_w_Tx*O_w_Tx*r_m1T)...
       - m*r_m2Tx*(T_a_m2T + 2*O_w_Tx*T_v_m2T + O_w_Tx*O_w_Tx*r_m2T)...
       - m*r_m3Tx*(T_a_m3T + 2*O_w_Tx*T_v_m3T + O_w_Tx*O_w_Tx*r_m3T)...
       - m*r_m4Tx*(T_a_m4T + 2*O_w_Tx*T_v_m4T + O_w_Tx*O_w_Tx*r_m4T)...
       - m*r_m5Tx*(T_a_m5T + 2*O_w_Tx*T_v_m5T + O_w_Tx*O_w_Tx*r_m5T)...
       - m*r_m6Tx*(T_a_m6T + 2*O_w_Tx*T_v_m6T + O_w_Tx*O_w_Tx*r_m6T)...
       + r_CMTx*T_c_O*FG + (mf + 6*m)*cross(T_c_O*r_PT, T_a_CMT + ...
         2*O_w_Tx*T_v_CMT + O_w_Tx*O_w_Tx*r_CMT) - T_c_O*cross(r_PT, FG) ...
        - T_c_O*cross(r_PT, FW);%- T_c_O*cross(r_PT, FR);
f3_v = inv(Amat)*Bvec;
M_hat = inv(Amat);

end

== matlab function extControlwithTCP/command filter based backstepper1/MATLAB Function1 ==
  data: eta1 input; eta1_dot output; eta2 input; alpha input; wc input; f1 input; K1 input
function eta1_dot = eta1_dot_calc(eta1, eta2, alpha, wc, f1, K1)
eta1_dot = -K1*(eta1) + f1*(wc - alpha) + f1*eta2;
end

== matlab function extControlwithTCP/command filter based backstepper1/MATLAB Function2 ==
  data: eta2 input; K2 input; f3_v input; f3_u input; eta2_dot output
function eta2_dot = eta2_dot_calc(eta2, K2,f3_v, f3_u)
eta2_dot = -K2*eta2 + (f3_u - f3_v);
end

== matlab function extControlwithTCP/command filter based backstepper1/Subsystem/MATLAB Function ==
  data: u input; f3_u output size=3; u_dot input; u_ddot input; states input; v_thres parameter; d parameter; R parameter; mu0 parameter; mf parameter; m parameter; Izz parameter; Iyy parameter; Ixx parameter; g parameter
function f3_u = f3u_calculator(u,u_dot,u_ddot,states,v_thres, d, R, mu0, mf, m, Izz, Iyy, Ixx, g)
I_T = [Ixx,0,0;0,Iyy,0;0,0,Izz];
r_m1T = [u(1);0;0];             T_v_m1T = [u_dot(1);0;0]; T_a_m1T = [u_ddot(1);0;0];
r_m2T = [-(d - u(1));0;0];      T_v_m2T = [u_dot(1);0;0]; T_a_m2T = [u_ddot(1);0;0];
r_m3T = [0;u(2);0];             T_v_m3T = [0;u_dot(2);0]; T_a_m3T = [0;u_ddot(2);0];
r_m4T = [0;-(d - u(2));0];      T_v_m4T = [0;u_dot(2);0]; T_a_m4T = [0;u_ddot(2);0];
r_m5T = [0;0;u(3)];             T_v_m5T = [0;0;u_dot(3)]; T_a_m5T = [0;0;u_ddot(3)];
r_m6T = [0;0;-(d - u(3))];      T_v_m6T = [0;0;u_dot(3)]; T_a_m6T = [0;0;u_ddot(3)];
r_CMT = m*(r_m1T + r_m2T + r_m3T + r_m4T + r_m5T + r_m6T)/(6*m+mf);
T_v_CMT = m*(T_v_m1T + T_v_m2T + T_v_m3T + T_v_m4T + T_v_m5T + T_v_m6T)/(6*m+mf);
T_a_CMT = m*(T_a_m1T + T_a_m2T + T_a_m3T + T_a_m4T + T_a_m5T + T_a_m6T)/(6*m+mf);
r_CMTx = Vx(r_CMT);r_m1Tx = Vx(r_m1T);r_m2Tx = Vx(r_m2T);r_m3Tx = Vx(r_m3T);
r_m4Tx = Vx(r_m4T);r_m5Tx = Vx(r_m5T);r_m6Tx = Vx(r_m6T);
q0 = states(10);q1=states(11);q2=states(12);q3=states(13);
T_c_O = [q0^2 + q1^2 - q2^2 - q3^2, 2*(q1*q2 + q0*q3), 2*(q1*q3 - q0*q2);...
       2*(q1*q2 - q0*q3), q0^2 - q1^2 + q2^2 - q3^2, 2*(q2*q3 + q0*q1);...
       2*(q1*q3 + q0*q2), 2*(q2*q3 - q0*q1), q0^2 - q1^2 - q2^2 + q3^2];
O_c_T = transpose(T_c_O);  
r_PT = [0;0;-R];
r_PTx = Vx([0;0;-R]);
O_w_T = [states(1);states(2);states(3)]; O_w_Tx =Vx(O_w_T);

O_vel_TO = Vx(O_c_T*O_w_T)*[0;0;R];
u_TO = O_vel_TO(1);
v_TO = O_vel_TO(2);

murr = mu0*tanh((u_TO^2 + v_TO^2)/v_thres); 
roll_rest_coeff = [1,0,-murr*u_TO/sqrt(u_TO^2 + v_TO^2);0,1,-murr*v_TO/sqrt(u_TO^2 + v_TO^2);0,0,1];
FG = [0;0;-(mf+6*m)*g];
FR  = -murr*norm(FG)/sqrt(u_TO^2 + v_TO^2)*[u_TO; v_TO; 0];

f3_u = zeros(3,1);
Amat = I_T + (mf + 6*m)*r_CMTx*T_c_O*r_PTx*O_c_T - m*r_m1Tx*r_m1Tx - m*r_m2Tx*r_m2Tx...
       - m*r_m3Tx*r_m3Tx - m*r_m4Tx*r_m4Tx - m*r_m5Tx*r_m5Tx - m*r_m6Tx*r_m6Tx...
       - (mf + 6*m)*Vx(T_c_O*r_PT)*Vx(T_c_O*r_PT) + (mf + 6*m)*Vx(T_c_O*r_PT)*r_CMTx;
  %some mistakes here. check again 
Bvec = -cross(O_w_T,I_T*O_w_T) - m*cross(r_m1T,2*O_w_Tx*T_v_m1T + O_w_Tx*O_w_Tx*r_m1T)...
       - m*r_m2Tx*(T_a_m2T + 2*O_w_Tx*T_v_m2T + O_w_Tx*O_w_Tx*r_m2T)...
       - m*r_m3Tx*(T_a_m3T + 2*O_w_Tx*T_v_m3T + O_w_Tx*O_w_Tx*r_m3T)...
       - m*r_m4Tx*(T_a_m4T + 2*O_w_Tx*T_v_m4T + O_w_Tx*O_w_Tx*r_m4T)...
       - m*r_m5Tx*(T_a_m5T + 2*O_w_Tx*T_v_m5T + O_w_Tx*O_w_Tx*r_m5T)...
       - m*r_m6Tx*(T_a_m6T + 2*O_w_Tx*T_v_m6T + O_w_Tx*O_w_Tx*r_m6T)...
       + r_CMTx*T_c_O*FG + (mf + 6*m)*cross(T_c_O*r_PT, T_a_CMT + ...
         2*O_w_Tx*T_v_CMT + O_w_Tx*O_w_Tx*r_CMT) - T_c_O*cross(r_PT, FG) ...
         - T_c_O*cross(r_PT, FR);
f3_u = inv(Amat)*Bvec;
end

== matlab function extControlwithTCP/command filter based backstepper1/Subsystem1/MATLAB Function ==
  data: u input; f3_u output size=3; u_dot input; u_ddot input; states input; FW input; v_thres parameter; d parameter; R parameter; mu0 parameter; mf parameter; m parameter; Izz parameter; Iyy parameter; Ixx parameter; g parameter
function f3_u = f3u_calculator(u,u_dot,u_ddot,states,FW,v_thres, d, R, mu0, mf, m, Izz, Iyy, Ixx, g)
I_T = [Ixx,0,0;0,Iyy,0;0,0,Izz];
r_m1T = [u(1);0;0];             T_v_m1T = [u_dot(1);0;0]; T_a_m1T = [u_ddot(1);0;0];
r_m2T = [-(d - u(1));0;0];      T_v_m2T = [u_dot(1);0;0]; T_a_m2T = [u_ddot(1);0;0];
r_m3T = [0;u(2);0];             T_v_m3T = [0;u_dot(2);0]; T_a_m3T = [0;u_ddot(2);0];
r_m4T = [0;-(d - u(2));0];      T_v_m4T = [0;u_dot(2);0]; T_a_m4T = [0;u_ddot(2);0];
r_m5T = [0;0;u(3)];             T_v_m5T = [0;0;u_dot(3)]; T_a_m5T = [0;0;u_ddot(3)];
r_m6T = [0;0;-(d - u(3))];      T_v_m6T = [0;0;u_dot(3)]; T_a_m6T = [0;0;u_ddot(3)];
r_CMT = m*(r_m1T + r_m2T + r_m3T + r_m4T + r_m5T + r_m6T)/(6*m+mf);
T_v_CMT = m*(T_v_m1T + T_v_m2T + T_v_m3T + T_v_m4T + T_v_m5T + T_v_m6T)/(6*m+mf);
T_a_CMT = m*(T_a_m1T + T_a_m2T + T_a_m3T + T_a_m4T + T_a_m5T + T_a_m6T)/(6*m+mf);
r_CMTx = Vx(r_CMT);r_m1Tx = Vx(r_m1T);r_m2Tx = Vx(r_m2T);r_m3Tx = Vx(r_m3T);
r_m4Tx = Vx(r_m4T);r_m5Tx = Vx(r_m5T);r_m6Tx = Vx(r_m6T);
q0 = states(10);q1=states(11);q2=states(12);q3=states(13);
T_c_O = [q0^2 + q1^2 - q2^2 - q3^2, 2*(q1*q2 + q0*q3), 2*(q1*q3 - q0*q2);...
       2*(q1*q2 - q0*q3), q0^2 - q1^2 + q2^2 - q3^2, 2*(q2*q3 + q0*q1);...
       2*(q1*q3 + q0*q2), 2*(q2*q3 - q0*q1), q0^2 - q1^2 - q2^2 + q3^2];
O_c_T = transpose(T_c_O);  
r_PT = [0;0;-R];
r_PTx = Vx([0;0;-R]);
O_w_T = [states(1);states(2);states(3)]; O_w_Tx =Vx(O_w_T);

O_vel_TO = Vx(O_c_T*O_w_T)*[0;0;R];
u_TO = O_vel_TO(1);
v_TO = O_vel_TO(2);

murr = mu0*tanh((u_TO^2 + v_TO^2)/v_thres); 
roll_rest_coeff = [1,0,-murr*u_TO/sqrt(u_TO^2 + v_TO^2);0,1,-murr*v_TO/sqrt(u_TO^2 + v_TO^2);0,0,1];
FG = [0;0;-(mf+6*m)*g];
FR  = -murr*norm(FG)/sqrt(u_TO^2 + v_TO^2)*[u_TO; v_TO; 0];

f3_u = zeros(3,1);
Amat = I_T + (mf + 6*m)*r_CMTx*T_c_O*r_PTx*O_c_T - m*r_m1Tx*r_m1Tx - m*r_m2Tx*r_m2Tx...
       - m*r_m3Tx*r_m3Tx - m*r_m4Tx*r_m4Tx - m*r_m5Tx*r_m5Tx - m*r_m6Tx*r_m6Tx...
       - (mf + 6*m)*Vx(T_c_O*r_PT)*Vx(T_c_O*r_PT) + (mf + 6*m)*Vx(T_c_O*r_PT)*r_CMTx;
  %some mistakes here. check again 
Bvec = -cross(O_w_T,I_T*O_w_T) - m*cross(r_m1T,2*O_w_Tx*T_v_m1T + O_w_Tx*O_w_Tx*r_m1T)...
       - m*r_m2Tx*(T_a_m2T + 2*O_w_Tx*T_v_m2T + O_w_Tx*O_w_Tx*r_m2T)...
       - m*r_m3Tx*(T_a_m3T + 2*O_w_Tx*T_v_m3T + O_w_Tx*O_w_Tx*r_m3T)...
       - m*r_m4Tx*(T_a_m4T + 2*O_w_Tx*T_v_m4T + O_w_Tx*O_w_Tx*r_m4T)...
       - m*r_m5Tx*(T_a_m5T + 2*O_w_Tx*T_v_m5T + O_w_Tx*O_w_Tx*r_m5T)...
       - m*r_m6Tx*(T_a_m6T + 2*O_w_Tx*T_v_m6T + O_w_Tx*O_w_Tx*r_m6T)...
       + r_CMTx*T_c_O*FG + (mf + 6*m)*cross(T_c_O*r_PT, T_a_CMT + ...
         2*O_w_Tx*T_v_CMT + O_w_Tx*O_w_Tx*r_CMT) - T_c_O*cross(r_PT, FG) ...
         - T_c_O*cross(r_PT, FW);%- T_c_O*cross(r_PT, FR);
f3_u = inv(Amat)*Bvec;
end

== matlab function extControlwithTCP/command filter based backstepper1/alpha calculator ==
  data: ref input size=3; alpha output size=3; ref_dot input; states input size=13; R parameter size=1; f1 output size=[3,3]; K1 output size=[3,3]
function [alpha, f1, K1] = alpha_calculator(ref, ref_dot, states, R)
q0 = states(10); q1 = states(11); q2 = states(12); q3 = states(13);

xc_dot = ref_dot;
xc = ref;
x = [states(7); states(8); states(9)];

K1 = 3*eye(3);

Rx = [0,R,0;-R,0,0;0,0,1];

T_c_O = [q0^2 + q1^2 - q2^2 - q3^2, 2*(q1*q2 + q0*q3), 2*(q1*q3 - q0*q2);...
2*(q1*q2 - q0*q3), q0^2 - q1^2 + q2^2 - q3^2, 2*(q2*q3 + q0*q1);...
2*(q1*q3 + q0*q2), 2*(q2*q3 - q0*q1), q0^2 - q1^2 - q2^2 + q3^2];
O_c_T = transpose(T_c_O);

f1 = Rx*O_c_T;
alpha = inv(f1)*(xc_dot - K1*(x - xc));
end

== matlab function extControlwithTCP/command filter based backstepper1/main one/MATLAB Function ==
  data: u input; f3_u output size=3; u_dot input; u_ddot input; states input; v_thres parameter; d parameter; R parameter; mu0 parameter; mf parameter; m parameter; Izz parameter; Iyy parameter; Ixx parameter; g parameter
function f3_u = f3u_calculator(u,u_dot,u_ddot,states,v_thres, d, R, mu0, mf, m, Izz, Iyy, Ixx, g)
I_T = [Ixx,0,0;0,Iyy,0;0,0,Izz];
r_m1T = [u(1);0;0];             T_v_m1T = [u_dot(1);0;0]; T_a_m1T = [u_ddot(1);0;0];
r_m2T = [-(d - u(1));0;0];      T_v_m2T = [u_dot(1);0;0]; T_a_m2T = [u_ddot(1);0;0];
r_m3T = [0;u(2);0];             T_v_m3T = [0;u_dot(2);0]; T_a_m3T = [0;u_ddot(2);0];
r_m4T = [0;-(d - u(2));0];      T_v_m4T = [0;u_dot(2);0]; T_a_m4T = [0;u_ddot(2);0];
r_m5T = [0;0;u(3)];             T_v_m5T = [0;0;u_dot(3)]; T_a_m5T = [0;0;u_ddot(3)];
r_m6T = [0;0;-(d - u(3))];      T_v_m6T = [0;0;u_dot(3)]; T_a_m6T = [0;0;u_ddot(3)];
r_CMT = m*(r_m1T + r_m2T + r_m3T + r_m4T + r_m5T + r_m6T)/(6*m+mf);
T_v_CMT = m*(T_v_m1T + T_v_m2T + T_v_m3T + T_v_m4T + T_v_m5T + T_v_m6T)/(6*m+mf);
T_a_CMT = m*(T_a_m1T + T_a_m2T + T_a_m3T + T_a_m4T + T_a_m5T + T_a_m6T)/(6*m+mf);
r_CMTx = Vx(r_CMT);r_m1Tx = Vx(r_m1T);r_m2Tx = Vx(r_m2T);r_m3Tx = Vx(r_m3T);
r_m4Tx = Vx(r_m4T);r_m5Tx = Vx(r_m5T);r_m6Tx = Vx(r_m6T);
q0 = states(10);q1=states(11);q2=states(12);q3=states(13);
T_c_O = [q0^2 + q1^2 - q2^2 - q3^2, 2*(q1*q2 + q0*q3), 2*(q1*q3 - q0*q2);...
       2*(q1*q2 - q0*q3), q0^2 - q1^2 + q2^2 - q3^2, 2*(q2*q3 + q0*q1);...
       2*(q1*q3 + q0*q2), 2*(q2*q3 - q0*q1), q0^2 - q1^2 - q2^2 + q3^2];
O_c_T = transpose(T_c_O);  
r_PT = [0;0;-R];
r_PTx = Vx([0;0;-R]);
O_w_T = [states(1);states(2);states(3)]; O_w_Tx =Vx(O_w_T);

O_vel_TO = Vx(O_c_T*O_w_T)*[0;0;R];
u_TO = O_vel_TO(1);
v_TO = O_vel_TO(2);

murr = mu0*tanh((u_TO^2 + v_TO^2)/v_thres); 
roll_rest_coeff = [1,0,-murr*u_TO/sqrt(u_TO^2 + v_TO^2);0,1,-murr*v_TO/sqrt(u_TO^2 + v_TO^2);0,0,1];
FG = [0;0;-(mf+6*m)*g];
FR  = -murr*norm(FG)/sqrt(u_TO^2 + v_TO^2)*[u_TO; v_TO; 0];

f3_u = zeros(3,1);
Amat = I_T + (mf + 6*m)*r_CMTx*T_c_O*r_PTx*O_c_T - m*r_m1Tx*r_m1Tx - m*r_m2Tx*r_m2Tx...
       - m*r_m3Tx*r_m3Tx - m*r_m4Tx*r_m4Tx - m*r_m5Tx*r_m5Tx - m*r_m6Tx*r_m6Tx...
       - (mf + 6*m)*Vx(T_c_O*r_PT)*Vx(T_c_O*r_PT) + (mf + 6*m)*Vx(T_c_O*r_PT)*r_CMTx;
  %some mistakes here. check again 
Bvec = -cross(O_w_T,I_T*O_w_T) - m*cross(r_m1T,2*O_w_Tx*T_v_m1T + O_w_Tx*O_w_Tx*r_m1T)...
       - m*r_m2Tx*(T_a_m2T + 2*O_w_Tx*T_v_m2T + O_w_Tx*O_w_Tx*r_m2T)...
       - m*r_m3Tx*(T_a_m3T + 2*O_w_Tx*T_v_m3T + O_w_Tx*O_w_Tx*r_m3T)...
       - m*r_m4Tx*(T_a_m4T + 2*O_w_Tx*T_v_m4T + O_w_Tx*O_w_Tx*r_m4T)...
       - m*r_m5Tx*(T_a_m5T + 2*O_w_Tx*T_v_m5T + O_w_Tx*O_w_Tx*r_m5T)...
       - m*r_m6Tx*(T_a_m6T + 2*O_w_Tx*T_v_m6T + O_w_Tx*O_w_Tx*r_m6T)...
       + r_CMTx*T_c_O*FG + (mf + 6*m)*cross(T_c_O*r_PT, T_a_CMT + ...
         2*O_w_Tx*T_v_CMT + O_w_Tx*O_w_Tx*r_CMT) - T_c_O*cross(r_PT, FG) ...
         ;%- T_c_O*cross(r_PT, FR);
f3_u = inv(Amat)*Bvec;
end
